simulink subsystem "discrete_PID_EF"  (R2024b)
settings: Solver=VariableStepAuto  StartTime=0.0  StopTime=10.0  RelTol=1e-3
values from neighbouring files (symbols this model uses):
  Kd = Kp*Td    (= 0.0676394167199)    [Controller_Discrete_Control_variables_25_04.m]    (also in Plant_EstimTrialUpdateLAB17_04_25.m = Kp*Td)
  Ki = Kp/Ti    (= 26.4286484862)    [Controller_Discrete_Control_variables_25_04.m]    (also in Plant_EstimTrialUpdateLAB17_04_25.m = Kp/Ti)
  Kp = 8.456047228584202    (= 8.45604722858)    [Controller_Discrete_Control_variables_25_04.m]    (also in Plant_EstimTrialUpdateLAB17_04_25.m = Dk*cos(Dphi))
  TL = 1/(2*wc)    (= 0.0165217010923)    [Controller_Discrete_Control_variables_25_04.m]    (also in Plant_EstimTrialUpdateLAB17_04_25.m = b * wc)
  Ts = Ts_values(2)    [A_final_measurements.m]    (also in Plant_EstimTrialUpdateLAB17_04_25.m = 0.001)
undefined symbols (not defined in the file or in its folder): DiscIntNeverNeededParam
settings Model: Creator=Riccardo Grosso  LastModifiedBy=Riccardo Grosso

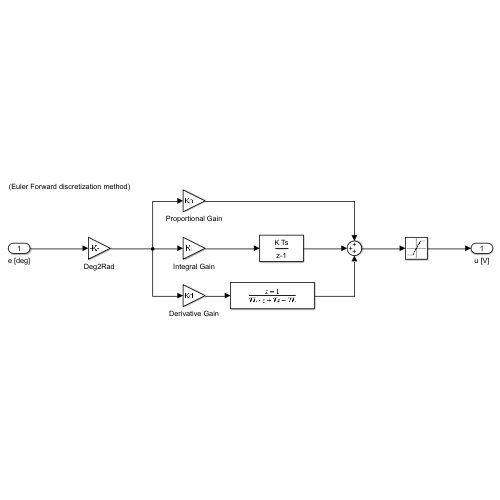
[thumbnail: Simulink's stored preview of the top-level diagram]
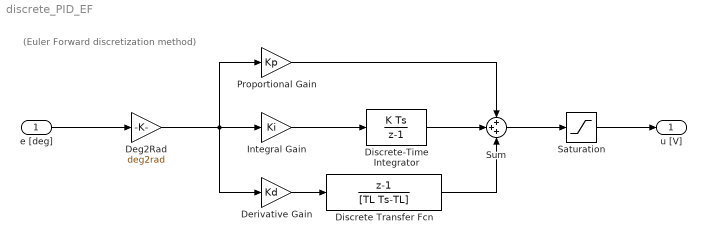
== system discrete_PID_EF ==
  note: (Euler Forward discretization method)
  e [deg] : Inport
  Deg2Rad : Gain  Gain=deg2rad
  Derivative Gain : Gain  Gain=Kd
  Discrete Transfer Fcn : DiscreteTransferFcn  Numerator=[1 -1]  Denominator=[TL Ts-TL]
  Discrete-Time Integrator : DiscreteIntegrator  SampleTime=Ts  ICPrevOutput=DiscIntNeverNeededParam  ICPrevScaledInput=DiscIntNeverNeededParam
  Integral Gain : Gain  Gain=Ki
  Proportional Gain : Gain  Gain=Kp
  Saturation : Saturate  UpperLimit=12  LowerLimit=-12
  Sum : Sum  Inputs=+++
  u [V] : Outport
  wires:
  Sum/1 -> Saturation/1
  Saturation/1 -> u [V]/1
  Discrete-Time Integrator/1 -> Sum/2
  Discrete Transfer Fcn/1 -> Sum/3
  Integral Gain/1 -> Discrete-Time Integrator/1
  Derivative Gain/1 -> Discrete Transfer Fcn/1
  Proportional Gain/1 -> Sum/1
  e [deg]/1 -> Deg2Rad/1
  Deg2Rad/1 -> Proportional Gain/1, Derivative Gain/1, Integral Gain/1
